simulink model "Observer"  (R2019b)
settings: Solver=VariableStepAuto  StartTime=0.0  StopTime=time_validation(end)  FixedStep=20e-3  RelTol=1e-3
values from neighbouring files (symbols this model uses):
  A = [-R_a/L_a, -c_e/L_a; c_m/J_m, 0]    [model_parameters.m]
  B = [k_p/L_a; 0]    [model_parameters.m]
  C = [0, 1]    [model_parameters.m]
  K = [k1_num; k2_num]    [Obtaining_observer.m]    (also in model_parameters.m = [-10.26; 331.50])
  tay = 64.453e-3    (= 0.064453)    [model_parameters.m]
settings Model: Creator=Олег  LastModifiedBy=Олег

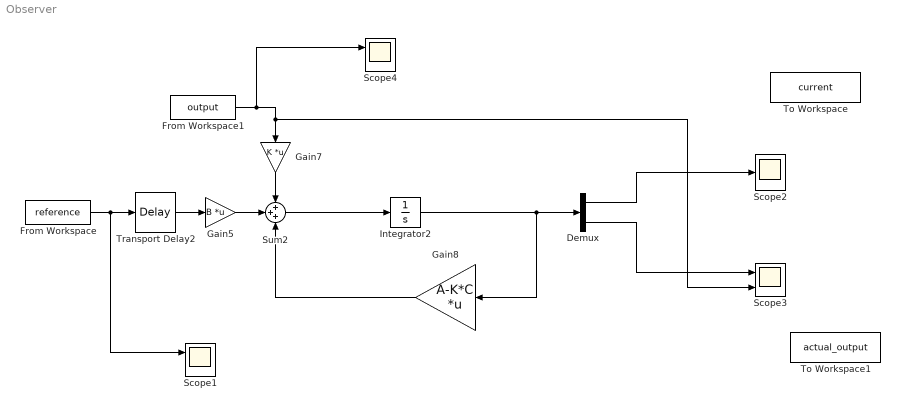
== system Observer ==
  Demux : Demux  Outputs=2
  From Workspace : FromWorkspace  VariableName=reference  OutputAfterFinalValue=Setting to zero
  From Workspace1 : FromWorkspace  VariableName=output  OutputAfterFinalValue=Setting to zero
  Gain5 : Gain  Gain=B  Multiplication=Matrix(K*u)
  Gain7 : Gain  Gain=K  Multiplication=Matrix(K*u)
  Gain8 : Gain  Gain=A-K*C  Multiplication=Matrix(K*u)
  Integrator2 : Integrator  InitialCondition=[0; 0]
  Scope1 : Scope  NumInputPorts=2
  Scope2 : Scope
  Scope3 : Scope  NumInputPorts=2
  Scope4 : Scope  NumInputPorts=2
  Sum2 : Sum  Inputs=+++
  To Workspace : ToWorkspace  VariableName=current  SaveFormat=Timeseries  SampleTime=-1
  To Workspace1 : ToWorkspace  VariableName=actual_output  SaveFormat=Timeseries  SampleTime=-1
  Transport Delay2 : TransportDelay  DelayTime=tay
  wires:
  Gain5/1 -> Sum2/2
  Gain8/1 -> Sum2/3
  Integrator2/1 -> Demux/1, Gain8/1
  Gain7/1 -> Sum2/1
  Sum2/1 -> Integrator2/1
  Transport Delay2/1 -> Gain5/1
  From Workspace/1 -> Scope1/1, Transport Delay2/1
  From Workspace1/1 -> Scope4/1, Scope3/2, Gain7/1
  Demux/1 -> Scope2/1
  Demux/2 -> Scope3/1
